simulink model "Propofol_Children"  (R2022a)
settings: Solver=FixedStepAuto  StartTime=0.0  StopTime=50  FixedStep=0.05  RelTol=1e-3
values from neighbouring files (symbols this model uses):
  delay = Patient(patient,11)    [LoadPatient.m]
  E0 = Patient(patient,9)    [LoadPatient.m]
  E50 = Patient(patient,13)    [LoadPatient.m]
  gamma = Patient(patient,14)    [LoadPatient.m]
  k = Patient(patient,12)    [LoadPatient.m]
  Kp = 0.58 * tau / (K * T)    [CalculaModelo.m]    (also in PlotAllPatients.m = -21.673)
  setpoint = set1    (= 52)    [PlotAllPatients.m]
libraries: slpidlib x1
settings Model: Creator=mluser  LastModifiedBy=phcs

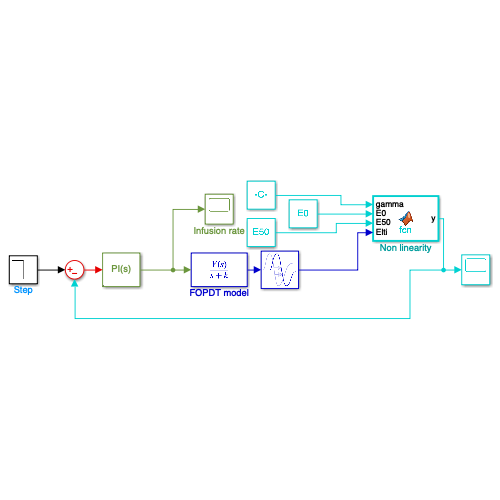
[thumbnail: Simulink's stored preview of the top-level diagram]
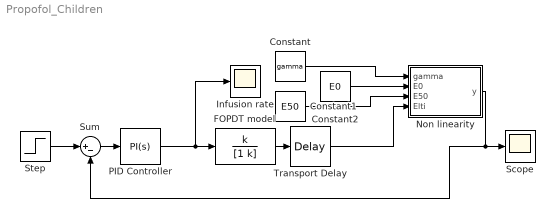
== system Propofol_Children ==
  Constant : Constant  Value=gamma
  Constant1 : Constant  Value=E50
  Constant2 : Constant  Value=E0
  FOPDT model : TransferFcn  Numerator=k  Denominator=[1 k]
  Infusion rate : Scope
  Non linearity : MATLAB Function  TreatAsAtomicUnit=on
  PID Controller : slpidlib/PID Controller  Controller=PI  Form=Parallel  TimeDomain=Continuous-time  UseExternalTs=off  SampleTime=-1  IntegratorMethod=Forward Euler  FilterMethod=Forward Euler  ControllerParametersSource=internal  P=Kp  I=Kp / Ti  UseKiTs=off  D=0  N=100  UseFilter=on  TunerSelectOption=Transfer Function Based (PID Tuner App)  InitialConditionSource=internal  InitialConditionForIntegrator=0  InitialConditionForFilter=0  DifferentiatorICPrevScaledInput=0  ExternalReset=none  TrackingMode=off  Kt=1  LimitOutput=off  SatLimitsSource=internal  UpperSaturationLimit=inf  LowerSaturationLimit=-inf  LinearizeAsGain=on  AntiWindupMode=none  Kb=1  POutMin=[]  POutMax=[]  IOutMin=[]  IOutMax=[]  DOutMin=[]  DOutMax=[]  NOutMin=[]  NOutMax=[]  SumOutMin=[]  SumOutMax=[]  SaturationOutMin=[]  SaturationOutMax=[]  PParamMin=[]  PParamMax=[]  IParamMin=[]  IParamMax=[]  DParamMin=[]  DParamMax=[]  NParamMin=[]  NParamMax=[]  KbParamMin=[]  KbParamMax=[]  KtParamMin=[]  KtParamMax=[]  KbOutMin=[]  KbOutMax=[]  KtOutMin=[]  KtOutMax=[]  IntegratorOutMin=[]  IntegratorOutMax=[]  FilterOutMin=[]  FilterOutMax=[]  SumI1OutMin=[]  SumI1OutMax=[]  SumI2OutMin=[]  SumI2OutMax=[]  SumI3OutMin=[]  SumI3OutMax=[]  SumI4OutMin=[]  SumI4OutMax=[]  SumDOutMin=[]  SumDOutMax=[]  DifferentiatorOutMin=[]  DifferentiatorOutMax=[]  FilterDiffOutCoefMin=[]  FilterDiffOutCoefMax=[]  ReciprocalOutMin=[]  ReciprocalOutMax=[]  SumDenOutMin=[]  SumDenOutMax=[]  SumNumOutMin=[]  SumNumOutMax=[]  DivideOutMin=[]  DivideOutMax=[]  UdiffTsProdOutMin=[]  UdiffTsProdOutMax=[]  NTsProdOutMin=[]  NTsProdOutMax=[]  UintegralTsProdOutMin=[]  UintegralTsProdOutMax=[]  UngainTsProdOutMin=[]  UngainTsProdOutMax=[]  IntegratorContinuousStateAttributes=''  IntegratorStateMustResolveToSignalObject=off  IntegratorRTWStateStorageClass=Auto  FilterContinuousStateAttributes=''  FilterStateMustResolveToSignalObject=off  FilterRTWStateStorageClass=Auto  ParallelPVariant=InternalParameters  IdealPVariant=Disabled  IVariant=InternalParameters  DVariant=Disabled  IntegratorVariant=Continuous  SatVariant=Disabled  AWVariant=Passthrough  PCopyVariant=Disabled  TRVariant=Disabled  FdbkBlocksVariant=Forward  IdealPFdbkVariant=Disabled  SatFdbkVariant=Disabled  DerivativeFilterVariant=Disabled  NVariant=Disabled  NCopyVariant=Disabled_SignalSpec  FilterICVariant=Disabled  IntegratorICVariant=InternalICs  ExternalResetVariant=Disabled  TRSumVariant=Passthrough  SumFdbkVariant=Disabled  SumVariant=Sum_PI  TsampFilterVariant=InternalTs  TsampNgainVariant=Passthrough  TsampIntegralVariant=Passthrough  ExternalSaturationOutDataTypeStr=Inherit: Same as second input  aMode=0
  Scope : Scope
  Step : Step  Time=0  Before=E0  After=setpoint  SampleTime=0
  Sum : Sum  Inputs=|+-
  Transport Delay : TransportDelay  DelayTime=delay/60
  wires:
  FOPDT model/1 -> Transport Delay/1
  PID Controller/1 -> Infusion rate/1, FOPDT model/1
  Non linearity/1(y) -> Sum/2, Scope/1
  Constant2/1 -> Non linearity/2(E0)
  Constant1/1 -> Non linearity/3(E50)
  Constant/1 -> Non linearity/1(gamma)
  Transport Delay/1 -> Non linearity/4(Elti)
  Sum/1 -> PID Controller/1
  Step/1 -> Sum/1

== matlab function Propofol_Children/Non linearity ==
  data: gamma input; y output; E0 input; E50 input; Elti input
function y = fcn(gamma,E0,E50,Elti)

y = E0-E0*Elti^gamma/(E50^gamma+Elti^gamma);
